simulink model "PMAC_sim"  (R2019b)
settings: Solver=VariableStepAuto  StartTime=0.0  StopTime=1  MaxStep=10e-6  RelTol=1e-3
values from neighbouring files (symbols this model uses):
  Bm = 15.1e-4    (= 0.00151)    [LAB_FOCIM_sim.m]    (also in LABprep.m; PMAC_machine.m = 7.59908877318e-07; WK1L1_DCmachine.m = Bm_init + Tmax*(i/10)*0.01; WK2_InductionMachine.m = 0.0337986596081)
  J = 27.6e-3    (= 0.0276)    [LAB_FOCIM_sim.m]    (also in LABprep.m; PMAC_machine.m = 2.55e-08; WK1L1_DCmachine.m = 0.134; WK2_InductionMachine.m = 0.0068)
  lambda_m = 3.49e-3    (= 0.00349)    [PMAC_machine.m]
  Ld = Lq    (= 7.2e-05)    [PMAC_machine.m]
  Lq = Lls + Lm    (= 7.2e-05)    [PMAC_machine.m]
  omega = f*2*pi    (= 376991.118431)    [PMAC_machine.m]
  P = 2    [LAB_FOCIM_sim.m]    (also in PMAC_machine.m; WK2_InductionMachine.m; WK2_InductionMachine_LAB.m; WK4_FOCIM_mScript.m)
  r_s = 1.3    [PMAC_machine.m]
  T_load = 0    [PMAC_machine.m]
  Vmax = 230    [LAB_FOCIM_sim.m]    (also in PMAC_machine.m = 24; WK2_InductionMachine.m; WK2_InductionMachine_LAB.m; WK4_FOCIM_mScript.m)
libraries: simulink x1
settings Model: Creator=Job  LastModifiedBy=Job

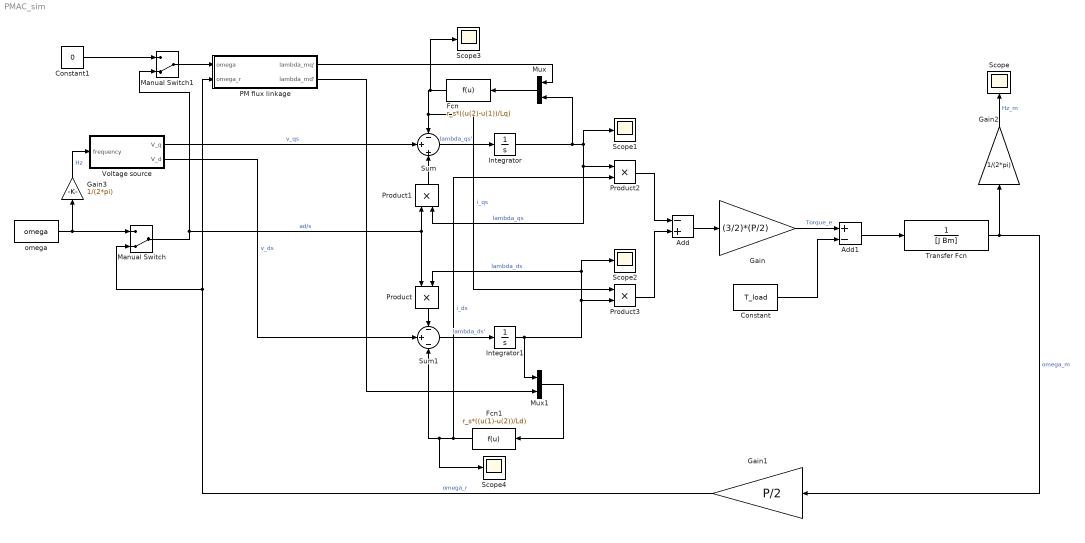
== system PMAC_sim ==
  Add : Sum  Inputs=-+
  Add1 : Sum  Inputs=+-
  Constant : Constant  Value=T_load
  Constant1 : Constant  Value=0
  Fcn : Fcn  Expr=r_s*((u(2)-u(1))/Lq)
  Fcn1 : Fcn  Expr=r_s*((u(1)-u(2))/Ld)
  Gain : Gain  Gain=(3/2)*(P/2)
  Gain1 : Gain  Gain=P/2
  Gain2 : Gain  Gain=1/(2*pi)
  Gain3 : Gain  Gain=1/(2*pi)
  Integrator : Integrator
  Integrator1 : Integrator
  Manual Switch : ManualSwitch  CurrentSetting=0
  Manual Switch1 : ManualSwitch  CurrentSetting=0
  Mux : Mux  Inputs=2
  Mux1 : Mux  Inputs=2
  PM flux linkage : Subsystem
  Product{,1..3} (4 alike) : Product
  Scope{,1..4} (5 alike) : Scope
  Sum : Sum  Inputs=-|+|+
  Sum1 : Sum  Inputs=-|+|-
  Transfer Fcn : TransferFcn  Denominator=[J Bm]
  Voltage source : Subsystem
  omega : Constant  Value=omega
  wires:
  Sum/1 -> Integrator/1  "lambda_qs'"
  Sum1/1 -> Integrator1/1  "lambda_ds'"
  Integrator/1 -> Mux/2, Scope1/1, Product2/1, Product1/2  "lambda_qs"
  Integrator1/1 -> Mux1/1, Product3/2, Scope2/1, Product/2  "lambda_ds"
  Product1/1 -> Sum/3
  Manual Switch/1 -> Manual Switch1/2, Product1/1, Product/1  "ad/s"
  Product/1 -> Sum1/1
  Voltage source/1(V_q) -> Sum/2  "v_qs"
  Voltage source/2(V_d) -> Sum1/2  "v_ds"
  PM flux linkage/1(lambda_mq') -> Mux/1
  Mux/1 -> Fcn/1
  Fcn/1 -> Scope3/1, Product3/1, Sum/1  "i_qs"
  PM flux linkage/2(lambda_md') -> Mux1/2
  Fcn1/1 -> Product2/2, Scope4/1, Sum1/3  "i_ds"
  Mux1/1 -> Fcn1/1
  Product2/1 -> Add/1
  Product3/1 -> Add/2
  Add/1 -> Gain/1
  Gain/1 -> Add1/1  "Torque_e"
  Transfer Fcn/1 -> Gain2/1, Gain1/1  "omega_m"
  Constant/1 -> Add1/2
  Add1/1 -> Transfer Fcn/1
  Gain1/1 -> PM flux linkage/2(omega_r), Manual Switch/2  "omega_r"
  Gain2/1 -> Scope/1  "Hz_m"
  omega/1 -> Gain3/1, Manual Switch/1
  Gain3/1 -> Voltage source/1(frequency)  "Hz"
  Constant1/1 -> Manual Switch1/1
  Manual Switch1/1 -> PM flux linkage/1(omega)

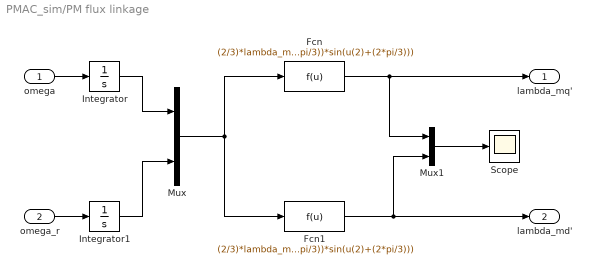
== system PMAC_sim/PM flux linkage ==
  omega : Inport
  omega_r : Inport  Port=2
  Fcn : Fcn  Expr=(2/3)*lambda_m*(cos(u(1))*sin(u(2))+cos(u(1)-(2*pi/3))*sin(u(2)-(2*pi/3))+cos(u(1)+(2*pi/3))*sin(u(2)+(2*pi/3)))
  Fcn1 : Fcn  Expr=(2/3)*lambda_m*(sin(u(1))*sin(u(2))+sin(u(1)-(2*pi/3))*sin(u(2)-(2*pi/3))+sin(u(1)+(2*pi/3))*sin(u(2)+(2*pi/3)))
  Integrator : Integrator
  Integrator1 : Integrator
  Mux : Mux  Inputs=2
  Mux1 : Mux  Inputs=2
  Scope : Scope
  lambda_mq' : Outport
  lambda_md' : Outport  Port=2
  wires:
  omega/1 -> Integrator/1
  omega_r/1 -> Integrator1/1
  Integrator1/1 -> Mux/2
  Integrator/1 -> Mux/1
  Fcn1/1 -> Mux1/2, lambda_md'/1
  Fcn/1 -> Mux1/1, lambda_mq'/1
  Mux/1 -> Fcn1/1, Fcn/1
  Mux1/1 -> Scope/1

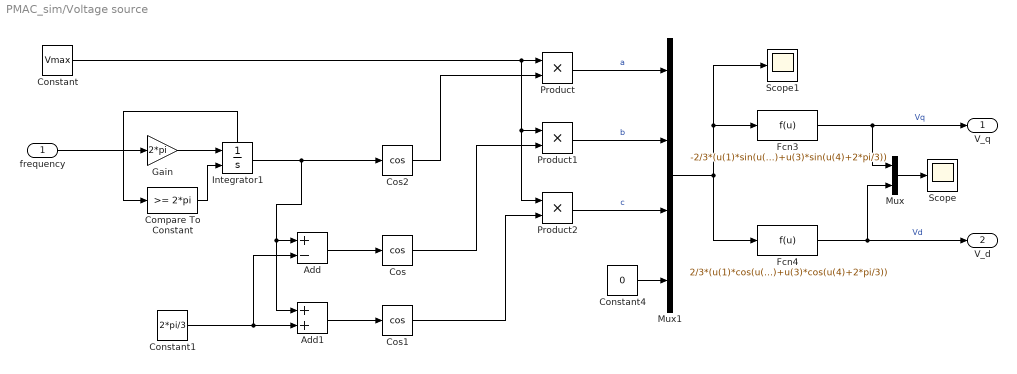
== system PMAC_sim/Voltage source ==
  frequency : Inport
  Add : Sum  Inputs=+-
  Add1 : Sum
  Compare To Constant : simulink/Logic and Bit Operations/Compare To Constant  relop=>=  const=2*pi  OutDataTypeStr=boolean
  Constant : Constant  Value=Vmax
  Constant1 : Constant  Value=2*pi/3
  Constant4 : Constant  Value=0
  Cos : Trigonometry  Operator=cos
  Cos1 : Trigonometry  Operator=cos
  Cos2 : Trigonometry  Operator=cos
  Fcn3 : Fcn  Expr=-2/3*(u(1)*sin(u(4))+u(2)*sin(u(4)-2*pi/3)+u(3)*sin(u(4)+2*pi/3))
  Fcn4 : Fcn  Expr=2/3*(u(1)*cos(u(4))+u(2)*cos(u(4)-2*pi/3)+u(3)*cos(u(4)+2*pi/3))
  Gain : Gain  Gain=2*pi
  Integrator1 : Integrator  ExternalReset=rising  ShowStatePort=on
  Mux : Mux  Inputs=2
  Mux1 : Mux
  Product : Product
  Product1 : Product
  Product2 : Product
  Scope : Scope
  Scope1 : Scope
  V_q : Outport
  V_d : Outport  Port=2
  wires:
  Fcn4/1 -> Mux/2, V_d/1  "Vd"
  Constant/1 -> Product1/1, Product2/1, Product/1
  Product/1 -> Mux1/1  "a"
  Constant1/1 -> Add/2, Add1/2
  Cos/1 -> Product1/2
  Product2/1 -> Mux1/3  "c"
  Fcn3/1 -> Mux/1, V_q/1  "Vq"
  Compare To Constant/1 -> Integrator1/2
  Product1/1 -> Mux1/2  "b"
  Gain/1 -> Integrator1/1
  Add1/1 -> Cos1/1
  Cos1/1 -> Product2/2
  Add/1 -> Cos/1
  Cos2/1 -> Product/2
  Integrator1/1 -> Cos2/1, Add1/1, Add/1
  Constant4/1 -> Mux1/4
  Integrator1/State -> Compare To Constant/1
  frequency/1 -> Gain/1
  Mux/1 -> Scope/1
  Mux1/1 -> Fcn4/1, Scope1/1, Fcn3/1
